simulink model "test_mdl_NI"  (R2018a)
settings: Solver=VariableStepAuto  StartTime=0.0  StopTime=10.0  RelTol=1e-3
(part 20 of 24)

== system test_mdl_NI/CAN_Signal/GWM/Other_GWMTx/PreCond_Hev_Data2_FD1 ==
  in : Inport
  BattTracClntFlw_Pc_Rq : Subsystem
  BattTrac_I_EstVsc : Subsystem
  DrvCondTpRrDefrs_B_Rq : Subsystem
  HtrnAin_UHi_Actl : Subsystem
  HtrnHvilOpen_B_Actl : Subsystem
  HtrnMil_D_Rq : Subsystem
  HtrnOvrTeLamp_B_Dsply : Subsystem
  HtrnSrvcRqd_B_Dsply : Subsystem
  PreCondActv_B_Actl : Subsystem
  PtWakeupDeltaT_T_Rq : Subsystem
  bus_creator : BusCreator  Inputs=10
  bus_selector : BusSelector  OutputSignals=BattTracClntFlw_Pc_Rq,BattTrac_I_EstVsc,DrvCondTpRrDefrs_B_Rq,HtrnAin_UHi_Actl,HtrnHvilOpen_B_Actl,HtrnMil_D_Rq,HtrnOvrTeLamp_B_Dsply,HtrnSrvcRqd_B_Dsply,PreCondActv_B_Actl,PtWakeupDeltaT_T_Rq
  out_port : Outport
  wires:
  bus_creator/1 -> out_port/1  "PreCond_Hev_Data2_FD1"
  BattTracClntFlw_Pc_Rq/1(out) -> bus_creator/1  "BattTracClntFlw_Pc_Rq"
  BattTrac_I_EstVsc/1(out) -> bus_creator/2  "BattTrac_I_EstVsc"
  DrvCondTpRrDefrs_B_Rq/1(out) -> bus_creator/3  "DrvCondTpRrDefrs_B_Rq"
  HtrnAin_UHi_Actl/1(out) -> bus_creator/4  "HtrnAin_UHi_Actl"
  HtrnHvilOpen_B_Actl/1(out) -> bus_creator/5  "HtrnHvilOpen_B_Actl"
  HtrnMil_D_Rq/1(out) -> bus_creator/6  "HtrnMil_D_Rq"
  HtrnOvrTeLamp_B_Dsply/1(out) -> bus_creator/7  "HtrnOvrTeLamp_B_Dsply"
  HtrnSrvcRqd_B_Dsply/1(out) -> bus_creator/8  "HtrnSrvcRqd_B_Dsply"
  PreCondActv_B_Actl/1(out) -> bus_creator/9  "PreCondActv_B_Actl"
  PtWakeupDeltaT_T_Rq/1(out) -> bus_creator/10  "PtWakeupDeltaT_T_Rq"
  bus_selector/1 -> BattTracClntFlw_Pc_Rq/1(in)  "<BattTracClntFlw_Pc_Rq>"
  bus_selector/2 -> BattTrac_I_EstVsc/1(in)  "<BattTrac_I_EstVsc>"
  bus_selector/3 -> DrvCondTpRrDefrs_B_Rq/1(in)  "<DrvCondTpRrDefrs_B_Rq>"
  bus_selector/4 -> HtrnAin_UHi_Actl/1(in)  "<HtrnAin_UHi_Actl>"
  bus_selector/5 -> HtrnHvilOpen_B_Actl/1(in)  "<HtrnHvilOpen_B_Actl>"
  bus_selector/6 -> HtrnMil_D_Rq/1(in)  "<HtrnMil_D_Rq>"
  bus_selector/7 -> HtrnOvrTeLamp_B_Dsply/1(in)  "<HtrnOvrTeLamp_B_Dsply>"
  bus_selector/8 -> HtrnSrvcRqd_B_Dsply/1(in)  "<HtrnSrvcRqd_B_Dsply>"
  bus_selector/9 -> PreCondActv_B_Actl/1(in)  "<PreCondActv_B_Actl>"
  bus_selector/10 -> PtWakeupDeltaT_T_Rq/1(in)  "<PtWakeupDeltaT_T_Rq>"
  in/1 -> bus_selector/1

== system test_mdl_NI/CAN_Signal/GWM/Other_GWMTx/Suspension_Data_FD1 ==
  in : Inport
  SuspClkSync_No_Rq : Subsystem
  SuspFrntRight_L_Actl : Subsystem
  SuspFrnt_L_Actl : Subsystem
  SuspFrnt_L_Prev : Subsystem
  SuspRearRight_L_Actl : Subsystem
  SuspRear_L_Actl : Subsystem
  SuspRear_L_Prev : Subsystem
  bus_creator : BusCreator  Inputs=7
  bus_selector : BusSelector  OutputSignals=SuspClkSync_No_Rq,SuspFrntRight_L_Actl,SuspFrnt_L_Actl,SuspFrnt_L_Prev,SuspRearRight_L_Actl,SuspRear_L_Actl,SuspRear_L_Prev
  out_port : Outport
  wires:
  bus_creator/1 -> out_port/1  "Suspension_Data_FD1"
  SuspClkSync_No_Rq/1(out) -> bus_creator/1  "SuspClkSync_No_Rq"
  SuspFrntRight_L_Actl/1(out) -> bus_creator/2  "SuspFrntRight_L_Actl"
  SuspFrnt_L_Actl/1(out) -> bus_creator/3  "SuspFrnt_L_Actl"
  SuspFrnt_L_Prev/1(out) -> bus_creator/4  "SuspFrnt_L_Prev"
  SuspRearRight_L_Actl/1(out) -> bus_creator/5  "SuspRearRight_L_Actl"
  SuspRear_L_Actl/1(out) -> bus_creator/6  "SuspRear_L_Actl"
  SuspRear_L_Prev/1(out) -> bus_creator/7  "SuspRear_L_Prev"
  bus_selector/1 -> SuspClkSync_No_Rq/1(in)  "<SuspClkSync_No_Rq>"
  bus_selector/2 -> SuspFrntRight_L_Actl/1(in)  "<SuspFrntRight_L_Actl>"
  bus_selector/3 -> SuspFrnt_L_Actl/1(in)  "<SuspFrnt_L_Actl>"
  bus_selector/4 -> SuspFrnt_L_Prev/1(in)  "<SuspFrnt_L_Prev>"
  bus_selector/5 -> SuspRearRight_L_Actl/1(in)  "<SuspRearRight_L_Actl>"
  bus_selector/6 -> SuspRear_L_Actl/1(in)  "<SuspRear_L_Actl>"
  bus_selector/7 -> SuspRear_L_Prev/1(in)  "<SuspRear_L_Prev>"
  in/1 -> bus_selector/1

== system test_mdl_NI/CAN_Signal/GWM/Other_GWMTx/TesterPhysicalResGWM_FD1 ==
  in : Inport
  TesterPhysicalResGWM_F1 : Subsystem
  bus_creator : BusCreator  Inputs=1
  bus_selector : BusSelector  OutputSignals=TesterPhysicalResGWM_F1
  out_port : Outport
  wires:
  bus_creator/1 -> out_port/1  "TesterPhysicalResGWM_FD1"
  TesterPhysicalResGWM_F1/1(out) -> bus_creator/1  "TesterPhysicalResGWM_F1"
  bus_selector/1 -> TesterPhysicalResGWM_F1/1(in)  "<TesterPhysicalResGWM_F1>"
  in/1 -> bus_selector/1

== system test_mdl_NI/CAN_Signal/GWM/Other_GWMTx/TrailerAid_Data_FD1 ==
  in : Inport
  TrlBrkInitOut_D_Rq : Subsystem
  TrlrAidEnbl_D_Rq : Subsystem
  TrlrAidSetup_D_Rq : Subsystem
  TrlrAnOffstDir_D_Mem : Subsystem
  TrlrAnOffst_An_Mem : Subsystem
  TrlrAxleToBmpr_L_Actl : Subsystem
  TrlrBallToBmpr_L_Actl : Subsystem
  TrlrId_No_Actl : Subsystem
  TrlrRvrseCancl_B_Rq : Subsystem
  TrlrTrgtOffst_L_Actl : Subsystem
  TrlrTrgtPtrnId_No_Mem : Subsystem
  TrlrTrgtToBmpr_L_Actl : Subsystem
  bus_creator : BusCreator  Inputs=12
  bus_selector : BusSelector  OutputSignals=TrlBrkInitOut_D_Rq,TrlrAidEnbl_D_Rq,TrlrAidSetup_D_Rq,TrlrAnOffstDir_D_Mem,TrlrAnOffst_An_Mem,TrlrAxleToBmpr_L_Actl,TrlrBallToBmpr_L_Actl,TrlrId_No_Actl,TrlrRvrseCancl_B_Rq,TrlrTrgtOffst_L_Actl,TrlrTrgtPtrnId_No_Mem,TrlrTrgtToBmpr_L_Actl
  out_port : Outport
  wires:
  bus_creator/1 -> out_port/1  "TrailerAid_Data_FD1"
  TrlBrkInitOut_D_Rq/1(out) -> bus_creator/1  "TrlBrkInitOut_D_Rq"
  TrlrAidEnbl_D_Rq/1(out) -> bus_creator/2  "TrlrAidEnbl_D_Rq"
  TrlrAidSetup_D_Rq/1(out) -> bus_creator/3  "TrlrAidSetup_D_Rq"
  TrlrAnOffstDir_D_Mem/1(out) -> bus_creator/4  "TrlrAnOffstDir_D_Mem"
  TrlrAnOffst_An_Mem/1(out) -> bus_creator/5  "TrlrAnOffst_An_Mem"
  TrlrAxleToBmpr_L_Actl/1(out) -> bus_creator/6  "TrlrAxleToBmpr_L_Actl"
  TrlrBallToBmpr_L_Actl/1(out) -> bus_creator/7  "TrlrBallToBmpr_L_Actl"
  TrlrId_No_Actl/1(out) -> bus_creator/8  "TrlrId_No_Actl"
  TrlrRvrseCancl_B_Rq/1(out) -> bus_creator/9  "TrlrRvrseCancl_B_Rq"
  TrlrTrgtOffst_L_Actl/1(out) -> bus_creator/10  "TrlrTrgtOffst_L_Actl"
  TrlrTrgtPtrnId_No_Mem/1(out) -> bus_creator/11  "TrlrTrgtPtrnId_No_Mem"
  TrlrTrgtToBmpr_L_Actl/1(out) -> bus_creator/12  "TrlrTrgtToBmpr_L_Actl"
  bus_selector/1 -> TrlBrkInitOut_D_Rq/1(in)  "<TrlBrkInitOut_D_Rq>"
  bus_selector/2 -> TrlrAidEnbl_D_Rq/1(in)  "<TrlrAidEnbl_D_Rq>"
  bus_selector/3 -> TrlrAidSetup_D_Rq/1(in)  "<TrlrAidSetup_D_Rq>"
  bus_selector/4 -> TrlrAnOffstDir_D_Mem/1(in)  "<TrlrAnOffstDir_D_Mem>"
  bus_selector/5 -> TrlrAnOffst_An_Mem/1(in)  "<TrlrAnOffst_An_Mem>"
  bus_selector/6 -> TrlrAxleToBmpr_L_Actl/1(in)  "<TrlrAxleToBmpr_L_Actl>"
  bus_selector/7 -> TrlrBallToBmpr_L_Actl/1(in)  "<TrlrBallToBmpr_L_Actl>"
  bus_selector/8 -> TrlrId_No_Actl/1(in)  "<TrlrId_No_Actl>"
  bus_selector/9 -> TrlrRvrseCancl_B_Rq/1(in)  "<TrlrRvrseCancl_B_Rq>"
  bus_selector/10 -> TrlrTrgtOffst_L_Actl/1(in)  "<TrlrTrgtOffst_L_Actl>"
  bus_selector/11 -> TrlrTrgtPtrnId_No_Mem/1(in)  "<TrlrTrgtPtrnId_No_Mem>"
  bus_selector/12 -> TrlrTrgtToBmpr_L_Actl/1(in)  "<TrlrTrgtToBmpr_L_Actl>"
  in/1 -> bus_selector/1

== system test_mdl_NI/CAN_Signal/GWM/Other_GWMTx/TrailerAid_Stat1_FD1 ==
  in : Inport
  TrlrSnsId_No_Actl : Subsystem
  bus_creator : BusCreator  Inputs=1
  bus_selector : BusSelector  OutputSignals=TrlrSnsId_No_Actl
  out_port : Outport
  wires:
  bus_creator/1 -> out_port/1  "TrailerAid_Stat1_FD1"
  TrlrSnsId_No_Actl/1(out) -> bus_creator/1  "TrlrSnsId_No_Actl"
  bus_selector/1 -> TrlrSnsId_No_Actl/1(in)  "<TrlrSnsId_No_Actl>"
  in/1 -> bus_selector/1

== system test_mdl_NI/CAN_Signal/GWM/Other_GWMTx/TrailerAid_Stat2_FD1 ==
  in : Inport
  TrlrHitYaw_AnRate_Actl : Subsystem
  TrlrHitchYaw_An_Actl : Subsystem
  TrlrHitchYaw_D_Stat : Subsystem
  TrlrYawWActl_D_Qf : Subsystem
  TrlrYaw_W_Actl : Subsystem
  bus_creator : BusCreator  Inputs=5
  bus_selector : BusSelector  OutputSignals=TrlrHitYaw_AnRate_Actl,TrlrHitchYaw_An_Actl,TrlrHitchYaw_D_Stat,TrlrYawWActl_D_Qf,TrlrYaw_W_Actl
  out_port : Outport
  wires:
  bus_creator/1 -> out_port/1  "TrailerAid_Stat2_FD1"
  TrlrHitYaw_AnRate_Actl/1(out) -> bus_creator/1  "TrlrHitYaw_AnRate_Actl"
  TrlrHitchYaw_An_Actl/1(out) -> bus_creator/2  "TrlrHitchYaw_An_Actl"
  TrlrHitchYaw_D_Stat/1(out) -> bus_creator/3  "TrlrHitchYaw_D_Stat"
  TrlrYawWActl_D_Qf/1(out) -> bus_creator/4  "TrlrYawWActl_D_Qf"
  TrlrYaw_W_Actl/1(out) -> bus_creator/5  "TrlrYaw_W_Actl"
  bus_selector/1 -> TrlrHitYaw_AnRate_Actl/1(in)  "<TrlrHitYaw_AnRate_Actl>"
  bus_selector/2 -> TrlrHitchYaw_An_Actl/1(in)  "<TrlrHitchYaw_An_Actl>"
  bus_selector/3 -> TrlrHitchYaw_D_Stat/1(in)  "<TrlrHitchYaw_D_Stat>"
  bus_selector/4 -> TrlrYawWActl_D_Qf/1(in)  "<TrlrYawWActl_D_Qf>"
  bus_selector/5 -> TrlrYaw_W_Actl/1(in)  "<TrlrYaw_W_Actl>"
  in/1 -> bus_selector/1

== system test_mdl_NI/CAN_Signal/GWM/Other_GWMTx/TrailerBrakeInfo_FD1 ==
  in : Inport
  StopLamp_B_RqTrlrBrk : Subsystem
  TrlBrkInitOut_D_Stat : Subsystem
  TrlrBrkActCirct_B_Falt : Subsystem
  TrlrBrkActCnnct_B_Actl : Subsystem
  TrlrBrkCtl_B_Falt : Subsystem
  TrlrBrkDcnnt_B_Actl : Subsystem
  TrlrBrkDsply_B_Rq : Subsystem
  TrlrBrkGain_No_Actl : Subsystem
  TrlrBrkMde_D_Actl : Subsystem
  TrlrBrkOut_No_Dsply : Subsystem
  bus_creator : BusCreator  Inputs=10
  bus_selector : BusSelector  OutputSignals=StopLamp_B_RqTrlrBrk,TrlBrkInitOut_D_Stat,TrlrBrkActCirct_B_Falt,TrlrBrkActCnnct_B_Actl,TrlrBrkCtl_B_Falt,TrlrBrkDcnnt_B_Actl,TrlrBrkDsply_B_Rq,TrlrBrkGain_No_Actl,TrlrBrkMde_D_Actl,TrlrBrkOut_No_Dsply
  out_port : Outport
  wires:
  bus_creator/1 -> out_port/1  "TrailerBrakeInfo_FD1"
  StopLamp_B_RqTrlrBrk/1(out) -> bus_creator/1  "StopLamp_B_RqTrlrBrk"
  TrlBrkInitOut_D_Stat/1(out) -> bus_creator/2  "TrlBrkInitOut_D_Stat"
  TrlrBrkActCirct_B_Falt/1(out) -> bus_creator/3  "TrlrBrkActCirct_B_Falt"
  TrlrBrkActCnnct_B_Actl/1(out) -> bus_creator/4  "TrlrBrkActCnnct_B_Actl"
  TrlrBrkCtl_B_Falt/1(out) -> bus_creator/5  "TrlrBrkCtl_B_Falt"
  TrlrBrkDcnnt_B_Actl/1(out) -> bus_creator/6  "TrlrBrkDcnnt_B_Actl"
  TrlrBrkDsply_B_Rq/1(out) -> bus_creator/7  "TrlrBrkDsply_B_Rq"
  TrlrBrkGain_No_Actl/1(out) -> bus_creator/8  "TrlrBrkGain_No_Actl"
  TrlrBrkMde_D_Actl/1(out) -> bus_creator/9  "TrlrBrkMde_D_Actl"
  TrlrBrkOut_No_Dsply/1(out) -> bus_creator/10  "TrlrBrkOut_No_Dsply"
  bus_selector/1 -> StopLamp_B_RqTrlrBrk/1(in)  "<StopLamp_B_RqTrlrBrk>"
  bus_selector/2 -> TrlBrkInitOut_D_Stat/1(in)  "<TrlBrkInitOut_D_Stat>"
  bus_selector/3 -> TrlrBrkActCirct_B_Falt/1(in)  "<TrlrBrkActCirct_B_Falt>"
  bus_selector/4 -> TrlrBrkActCnnct_B_Actl/1(in)  "<TrlrBrkActCnnct_B_Actl>"
  bus_selector/5 -> TrlrBrkCtl_B_Falt/1(in)  "<TrlrBrkCtl_B_Falt>"
  bus_selector/6 -> TrlrBrkDcnnt_B_Actl/1(in)  "<TrlrBrkDcnnt_B_Actl>"
  bus_selector/7 -> TrlrBrkDsply_B_Rq/1(in)  "<TrlrBrkDsply_B_Rq>"
  bus_selector/8 -> TrlrBrkGain_No_Actl/1(in)  "<TrlrBrkGain_No_Actl>"
  bus_selector/9 -> TrlrBrkMde_D_Actl/1(in)  "<TrlrBrkMde_D_Actl>"
  bus_selector/10 -> TrlrBrkOut_No_Dsply/1(in)  "<TrlrBrkOut_No_Dsply>"
  in/1 -> bus_selector/1

== system test_mdl_NI/CAN_Signal/GWM/Other_GWMTx/TrailerInfo_2_FD1 ==
  in : Inport
  TrlrAidAn_URate_Actl : Subsystem
  TrlrAidAn_U_Actl : Subsystem
  TrlrAidCtl_U_RqDrv : Subsystem
  TrlrAidSwtch_D_RqDrv : Subsystem
  bus_creator : BusCreator  Inputs=4
  bus_selector : BusSelector  OutputSignals=TrlrAidAn_URate_Actl,TrlrAidAn_U_Actl,TrlrAidCtl_U_RqDrv,TrlrAidSwtch_D_RqDrv
  out_port : Outport
  wires:
  bus_creator/1 -> out_port/1  "TrailerInfo_2_FD1"
  TrlrAidAn_URate_Actl/1(out) -> bus_creator/1  "TrlrAidAn_URate_Actl"
  TrlrAidAn_U_Actl/1(out) -> bus_creator/2  "TrlrAidAn_U_Actl"
  TrlrAidCtl_U_RqDrv/1(out) -> bus_creator/3  "TrlrAidCtl_U_RqDrv"
  TrlrAidSwtch_D_RqDrv/1(out) -> bus_creator/4  "TrlrAidSwtch_D_RqDrv"
  bus_selector/1 -> TrlrAidAn_URate_Actl/1(in)  "<TrlrAidAn_URate_Actl>"
  bus_selector/2 -> TrlrAidAn_U_Actl/1(in)  "<TrlrAidAn_U_Actl>"
  bus_selector/3 -> TrlrAidCtl_U_RqDrv/1(in)  "<TrlrAidCtl_U_RqDrv>"
  bus_selector/4 -> TrlrAidSwtch_D_RqDrv/1(in)  "<TrlrAidSwtch_D_RqDrv>"
  in/1 -> bus_selector/1

== system test_mdl_NI/CAN_Signal/GWM/Other_GWMTx/TrailerInfo_FD1 ==
  in : Inport
  ParkLampTrlrOut_B_Stat : Subsystem
  StopLampTrlrOut_B_Stat : Subsystem
  TrlrBattChrg_D_Stat : Subsystem
  TrlrLampCnnct_B_Actl : Subsystem
  TrlrLampCtl_D_Stat : Subsystem
  TurnLampTrlrRl_B_Stat : Subsystem
  TurnLampTrlrRr_B_Stat : Subsystem
  bus_creator : BusCreator  Inputs=7
  bus_selector : BusSelector  OutputSignals=ParkLampTrlrOut_B_Stat,StopLampTrlrOut_B_Stat,TrlrBattChrg_D_Stat,TrlrLampCnnct_B_Actl,TrlrLampCtl_D_Stat,TurnLampTrlrRl_B_Stat,TurnLampTrlrRr_B_Stat
  out_port : Outport
  wires:
  bus_creator/1 -> out_port/1  "TrailerInfo_FD1"
  ParkLampTrlrOut_B_Stat/1(out) -> bus_creator/1  "ParkLampTrlrOut_B_Stat"
  StopLampTrlrOut_B_Stat/1(out) -> bus_creator/2  "StopLampTrlrOut_B_Stat"
  TrlrBattChrg_D_Stat/1(out) -> bus_creator/3  "TrlrBattChrg_D_Stat"
  TrlrLampCnnct_B_Actl/1(out) -> bus_creator/4  "TrlrLampCnnct_B_Actl"
  TrlrLampCtl_D_Stat/1(out) -> bus_creator/5  "TrlrLampCtl_D_Stat"
  TurnLampTrlrRl_B_Stat/1(out) -> bus_creator/6  "TurnLampTrlrRl_B_Stat"
  TurnLampTrlrRr_B_Stat/1(out) -> bus_creator/7  "TurnLampTrlrRr_B_Stat"
  bus_selector/1 -> ParkLampTrlrOut_B_Stat/1(in)  "<ParkLampTrlrOut_B_Stat>"
  bus_selector/2 -> StopLampTrlrOut_B_Stat/1(in)  "<StopLampTrlrOut_B_Stat>"
  bus_selector/3 -> TrlrBattChrg_D_Stat/1(in)  "<TrlrBattChrg_D_Stat>"
  bus_selector/4 -> TrlrLampCnnct_B_Actl/1(in)  "<TrlrLampCnnct_B_Actl>"
  bus_selector/5 -> TrlrLampCtl_D_Stat/1(in)  "<TrlrLampCtl_D_Stat>"
  bus_selector/6 -> TurnLampTrlrRl_B_Stat/1(in)  "<TurnLampTrlrRl_B_Stat>"
  bus_selector/7 -> TurnLampTrlrRr_B_Stat/1(in)  "<TurnLampTrlrRr_B_Stat>"
  in/1 -> bus_selector/1

== system test_mdl_NI/CAN_Signal/GWM/Other_GWMTx/VeyDynamics_Data_FD1 ==
  in : Inport
  AdptDrvMdeChassis_D_Rq : Subsystem
  AdptDrvMdePt_D_Rq : Subsystem
  AirSprngRateFl_D_Rq : Subsystem
  AirSprngRateFr_D_Rq : Subsystem
  AirSprngRateRl_D_Rq : Subsystem
  AirSprngRateRr_D_Rq : Subsystem
  AirSuspMsgTxt_D_Rq : Subsystem
  AirSusp_D_Stat : Subsystem
  BrkPadMsgTxt_D_Rq : Subsystem
  CcdMsgTxt_D_RqDsply : Subsystem
  Ccd_B_Falt : Subsystem
  SelDrvMdeSusp_D_Stat : Subsystem
  SuspDrvMde_D_Stat : Subsystem
  SuspType_B_Stat : Subsystem
  SuspVLim_B_Rq : Subsystem
  bus_creator : BusCreator  Inputs=15
  bus_selector : BusSelector  OutputSignals=AdptDrvMdeChassis_D_Rq,AdptDrvMdePt_D_Rq,AirSprngRateFl_D_Rq,AirSprngRateFr_D_Rq,AirSprngRateRl_D_Rq,AirSprngRateRr_D_Rq,AirSuspMsgTxt_D_Rq,AirSusp_D_Stat,BrkPadMsgTxt_D_Rq,CcdMsgTxt_D_RqDsply,Ccd_B_Falt,SelDrvMdeSusp_D_Stat,SuspDrvMde_D_Stat,SuspType_B_Stat,SuspVLim_B_Rq
  out_port : Outport
  wires:
  bus_creator/1 -> out_port/1  "VeyDynamics_Data_FD1"
  AdptDrvMdeChassis_D_Rq/1(out) -> bus_creator/1  "AdptDrvMdeChassis_D_Rq"
  AdptDrvMdePt_D_Rq/1(out) -> bus_creator/2  "AdptDrvMdePt_D_Rq"
  AirSprngRateFl_D_Rq/1(out) -> bus_creator/3  "AirSprngRateFl_D_Rq"
  AirSprngRateFr_D_Rq/1(out) -> bus_creator/4  "AirSprngRateFr_D_Rq"
  AirSprngRateRl_D_Rq/1(out) -> bus_creator/5  "AirSprngRateRl_D_Rq"
  AirSprngRateRr_D_Rq/1(out) -> bus_creator/6  "AirSprngRateRr_D_Rq"
  AirSuspMsgTxt_D_Rq/1(out) -> bus_creator/7  "AirSuspMsgTxt_D_Rq"
  AirSusp_D_Stat/1(out) -> bus_creator/8  "AirSusp_D_Stat"
  BrkPadMsgTxt_D_Rq/1(out) -> bus_creator/9  "BrkPadMsgTxt_D_Rq"
  CcdMsgTxt_D_RqDsply/1(out) -> bus_creator/10  "CcdMsgTxt_D_RqDsply"
  Ccd_B_Falt/1(out) -> bus_creator/11  "Ccd_B_Falt"
  SelDrvMdeSusp_D_Stat/1(out) -> bus_creator/12  "SelDrvMdeSusp_D_Stat"
  SuspDrvMde_D_Stat/1(out) -> bus_creator/13  "SuspDrvMde_D_Stat"
  SuspType_B_Stat/1(out) -> bus_creator/14  "SuspType_B_Stat"
  SuspVLim_B_Rq/1(out) -> bus_creator/15  "SuspVLim_B_Rq"
  bus_selector/1 -> AdptDrvMdeChassis_D_Rq/1(in)  "<AdptDrvMdeChassis_D_Rq>"
  bus_selector/2 -> AdptDrvMdePt_D_Rq/1(in)  "<AdptDrvMdePt_D_Rq>"
  bus_selector/3 -> AirSprngRateFl_D_Rq/1(in)  "<AirSprngRateFl_D_Rq>"
  bus_selector/4 -> AirSprngRateFr_D_Rq/1(in)  "<AirSprngRateFr_D_Rq>"
  bus_selector/5 -> AirSprngRateRl_D_Rq/1(in)  "<AirSprngRateRl_D_Rq>"
  bus_selector/6 -> AirSprngRateRr_D_Rq/1(in)  "<AirSprngRateRr_D_Rq>"
  bus_selector/7 -> AirSuspMsgTxt_D_Rq/1(in)  "<AirSuspMsgTxt_D_Rq>"
  bus_selector/8 -> AirSusp_D_Stat/1(in)  "<AirSusp_D_Stat>"
  bus_selector/9 -> BrkPadMsgTxt_D_Rq/1(in)  "<BrkPadMsgTxt_D_Rq>"
  bus_selector/10 -> CcdMsgTxt_D_RqDsply/1(in)  "<CcdMsgTxt_D_RqDsply>"
  bus_selector/11 -> Ccd_B_Falt/1(in)  "<Ccd_B_Falt>"
  bus_selector/12 -> SelDrvMdeSusp_D_Stat/1(in)  "<SelDrvMdeSusp_D_Stat>"
  bus_selector/13 -> SuspDrvMde_D_Stat/1(in)  "<SuspDrvMde_D_Stat>"
  bus_selector/14 -> SuspType_B_Stat/1(in)  "<SuspType_B_Stat>"
  bus_selector/15 -> SuspVLim_B_Rq/1(in)  "<SuspVLim_B_Rq>"
  in/1 -> bus_selector/1

== system test_mdl_NI/CAN_Signal/GWM/RCM/RCMSerialNumber_FD1_454 ==
  in : Inport
  RCMSerialNoByte1 : Subsystem
  RCMSerialNoByte2 : Subsystem
  RCMSerialNoByte3 : Subsystem
  RCMSerialNoByte4 : Subsystem
  RCMSerialNoByte5 : Subsystem
  RCMSerialNoByte6 : Subsystem
  RCMSerialNoByte7 : Subsystem
  RCMSerialNoByte8 : Subsystem
  bus_creator : BusCreator  Inputs=8
  bus_selector : BusSelector  OutputSignals=RCMSerialNoByte1,RCMSerialNoByte2,RCMSerialNoByte3,RCMSerialNoByte4,RCMSerialNoByte5,RCMSerialNoByte6,RCMSerialNoByte7,RCMSerialNoByte8
  out_port : Outport
  wires:
  bus_creator/1 -> out_port/1  "RCMSerialNumber_FD1_454"
  RCMSerialNoByte1/1(out) -> bus_creator/1  "RCMSerialNoByte1"
  RCMSerialNoByte2/1(out) -> bus_creator/2  "RCMSerialNoByte2"
  RCMSerialNoByte3/1(out) -> bus_creator/3  "RCMSerialNoByte3"
  RCMSerialNoByte4/1(out) -> bus_creator/4  "RCMSerialNoByte4"
  RCMSerialNoByte5/1(out) -> bus_creator/5  "RCMSerialNoByte5"
  RCMSerialNoByte6/1(out) -> bus_creator/6  "RCMSerialNoByte6"
  RCMSerialNoByte7/1(out) -> bus_creator/7  "RCMSerialNoByte7"
  RCMSerialNoByte8/1(out) -> bus_creator/8  "RCMSerialNoByte8"
  bus_selector/1 -> RCMSerialNoByte1/1(in)  "<RCMSerialNoByte1>"
  bus_selector/2 -> RCMSerialNoByte2/1(in)  "<RCMSerialNoByte2>"
  bus_selector/3 -> RCMSerialNoByte3/1(in)  "<RCMSerialNoByte3>"
  bus_selector/4 -> RCMSerialNoByte4/1(in)  "<RCMSerialNoByte4>"
  bus_selector/5 -> RCMSerialNoByte5/1(in)  "<RCMSerialNoByte5>"
  bus_selector/6 -> RCMSerialNoByte6/1(in)  "<RCMSerialNoByte6>"
  bus_selector/7 -> RCMSerialNoByte7/1(in)  "<RCMSerialNoByte7>"
  bus_selector/8 -> RCMSerialNoByte8/1(in)  "<RCMSerialNoByte8>"
  in/1 -> bus_selector/1

== system test_mdl_NI/CAN_Signal/GWM/RCM/RCMStatusMessage2_FD1_4C ==
  in : Inport
  EDRTriggerEvntSync : Subsystem
  FirstRowBuckleDriver : Subsystem
  FirstRowBuckleMid : Subsystem
  FirstRowBucklePsngr : Subsystem
  PassRstrnInd_Req : Subsystem
  PsngrFmidDetct_D_Actl : Subsystem
  PsngrFrntDetct_D_Actl : Subsystem
  RILReq : Subsystem
  RstrnImpactEvntStatus : Subsystem
  RstrnPsngrOn_D_Stat : Subsystem
  SecondRowBuckleDriver : Subsystem
  SecondRowBuckleMid : Subsystem
  SecondRowBucklePsngr : Subsystem
  ThirdRowBuckleDriver : Subsystem
  ThirdRowBuckleMid : Subsystem
  ThirdRowBucklePsngr : Subsystem
  bus_creator : BusCreator  Inputs=16
  bus_selector : BusSelector  OutputSignals=EDRTriggerEvntSync,FirstRowBuckleDriver,FirstRowBuckleMid,FirstRowBucklePsngr,PassRstrnInd_Req,PsngrFmidDetct_D_Actl,PsngrFrntDetct_D_Actl,RILReq,RstrnImpactEvntStatus,RstrnPsngrOn_D_Stat,SecondRowBuckleDriver,SecondRowBuckleMid,SecondRowBucklePsngr,ThirdRowBuckleDriver,ThirdRowBuckleMid,ThirdRowBucklePsngr
  out_port : Outport
  wires:
  bus_creator/1 -> out_port/1  "RCMStatusMessage2_FD1_4C"
  EDRTriggerEvntSync/1(out) -> bus_creator/1  "EDRTriggerEvntSync"
  FirstRowBuckleDriver/1(out) -> bus_creator/2  "FirstRowBuckleDriver"
  FirstRowBuckleMid/1(out) -> bus_creator/3  "FirstRowBuckleMid"
  FirstRowBucklePsngr/1(out) -> bus_creator/4  "FirstRowBucklePsngr"
  PassRstrnInd_Req/1(out) -> bus_creator/5  "PassRstrnInd_Req"
  PsngrFmidDetct_D_Actl/1(out) -> bus_creator/6  "PsngrFmidDetct_D_Actl"
  PsngrFrntDetct_D_Actl/1(out) -> bus_creator/7  "PsngrFrntDetct_D_Actl"
  RILReq/1(out) -> bus_creator/8  "RILReq"
  RstrnImpactEvntStatus/1(out) -> bus_creator/9  "RstrnImpactEvntStatus"
  RstrnPsngrOn_D_Stat/1(out) -> bus_creator/10  "RstrnPsngrOn_D_Stat"
  SecondRowBuckleDriver/1(out) -> bus_creator/11  "SecondRowBuckleDriver"
  SecondRowBuckleMid/1(out) -> bus_creator/12  "SecondRowBuckleMid"
  SecondRowBucklePsngr/1(out) -> bus_creator/13  "SecondRowBucklePsngr"
  ThirdRowBuckleDriver/1(out) -> bus_creator/14  "ThirdRowBuckleDriver"
  ThirdRowBuckleMid/1(out) -> bus_creator/15  "ThirdRowBuckleMid"
  ThirdRowBucklePsngr/1(out) -> bus_creator/16  "ThirdRowBucklePsngr"
  bus_selector/1 -> EDRTriggerEvntSync/1(in)  "<EDRTriggerEvntSync>"
  bus_selector/2 -> FirstRowBuckleDriver/1(in)  "<FirstRowBuckleDriver>"
  bus_selector/3 -> FirstRowBuckleMid/1(in)  "<FirstRowBuckleMid>"
  bus_selector/4 -> FirstRowBucklePsngr/1(in)  "<FirstRowBucklePsngr>"
  bus_selector/5 -> PassRstrnInd_Req/1(in)  "<PassRstrnInd_Req>"
  bus_selector/6 -> PsngrFmidDetct_D_Actl/1(in)  "<PsngrFmidDetct_D_Actl>"
  bus_selector/7 -> PsngrFrntDetct_D_Actl/1(in)  "<PsngrFrntDetct_D_Actl>"
  bus_selector/8 -> RILReq/1(in)  "<RILReq>"
  bus_selector/9 -> RstrnImpactEvntStatus/1(in)  "<RstrnImpactEvntStatus>"
  bus_selector/10 -> RstrnPsngrOn_D_Stat/1(in)  "<RstrnPsngrOn_D_Stat>"
  bus_selector/11 -> SecondRowBuckleDriver/1(in)  "<SecondRowBuckleDriver>"
  bus_selector/12 -> SecondRowBuckleMid/1(in)  "<SecondRowBuckleMid>"
  bus_selector/13 -> SecondRowBucklePsngr/1(in)  "<SecondRowBucklePsngr>"
  bus_selector/14 -> ThirdRowBuckleDriver/1(in)  "<ThirdRowBuckleDriver>"
  bus_selector/15 -> ThirdRowBuckleMid/1(in)  "<ThirdRowBuckleMid>"
  bus_selector/16 -> ThirdRowBucklePsngr/1(in)  "<ThirdRowBucklePsngr>"
  in/1 -> bus_selector/1

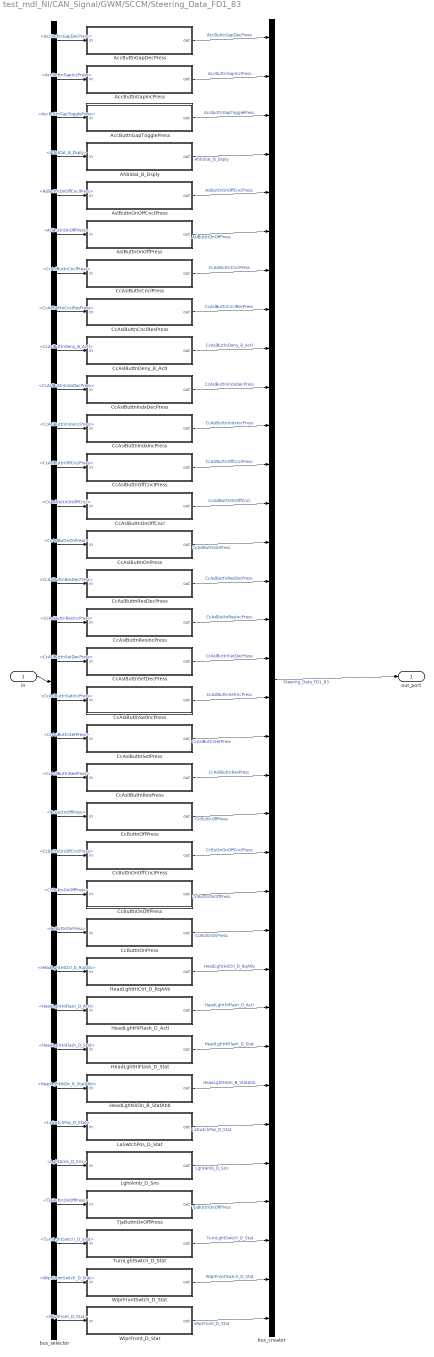
== system test_mdl_NI/CAN_Signal/GWM/SCCM/Steering_Data_FD1_83 ==
  in : Inport
  AccButtnGapDecPress : Subsystem
  AccButtnGapIncPress : Subsystem
  AccButtnGapTogglePress : Subsystem
  AhbStat_B_Dsply : Subsystem
  AslButtnOnOffCnclPress : Subsystem
  AslButtnOnOffPress : Subsystem
  CcAslButtnCnclPress : Subsystem
  CcAslButtnCnclResPress : Subsystem
  CcAslButtnDeny_B_Actl : Subsystem
  CcAslButtnIndxDecPress : Subsystem
  CcAslButtnIndxIncPress : Subsystem
  CcAslButtnOffCnclPress : Subsystem
  CcAslButtnOnOffCncl : Subsystem
  CcAslButtnOnPress : Subsystem
  CcAslButtnResDecPress : Subsystem
  CcAslButtnResIncPress : Subsystem
  CcAslButtnSetDecPress : Subsystem
  CcAslButtnSetIncPress : Subsystem
  CcAslButtnSetPress : Subsystem
  CcAsllButtnResPress : Subsystem
  CcButtnOffPress : Subsystem
  CcButtnOnOffCnclPress : Subsystem
  CcButtnOnOffPress : Subsystem
  CcButtnOnPress : Subsystem
  HeadLghtHiCtrl_D_RqAhb : Subsystem
  HeadLghtHiFlash_D_Actl : Subsystem
  HeadLghtHiFlash_D_Stat : Subsystem
  HeadLghtHiOn_B_StatAhb : Subsystem
  LaSwtchPos_D_Stat : Subsystem
  LghtAmb_D_Sns : Subsystem
  TjaButtnOnOffPress : Subsystem
  TurnLghtSwtch_D_Stat : Subsystem
  WiprFrontSwtch_D_Stat : Subsystem
  WiprFront_D_Stat : Subsystem
  bus_creator : BusCreator  Inputs=34
  bus_selector : BusSelector  OutputSignals=AccButtnGapDecPress,AccButtnGapIncPress,AccButtnGapTogglePress,AhbStat_B_Dsply,AslButtnOnOffCnclPress,AslButtnOnOffPress,CcAslButtnCnclPress,CcAslButtnCnclResPress,CcAslButtnDeny_B_Actl,CcAslButtnIndxDecPress,CcAslButtnIndxIncPress,CcAslButtnOffCnclPress,CcAslButtnOnOffCncl,CcAslButtnOnPress,CcAslButtnResDecPress,CcAslButtnResIncPress,CcAslButtnSetDecPress,CcAslButtnSetIncPress,CcAslButtnSetPress,CcAsllButtnResPress,CcButtnOffPress,CcButtnOnOffCnclPress,CcButtnOnOffPress,CcButtnOnPress,HeadLghtHiCtrl_D_RqAhb,HeadLghtHiFlash_D_Actl,HeadLghtHiFlash_D_Stat,HeadLghtHiOn_B_StatAhb,LaSwtchPos_D_Stat,LghtAmb_D_Sns,TjaButtnOnOffPress,TurnLghtSwtch_D_Stat,WiprFrontSwtch_D_Stat,WiprFront_D_Stat
  out_port : Outport
  wires:
  bus_creator/1 -> out_port/1  "Steering_Data_FD1_83"
  AccButtnGapDecPress/1(out) -> bus_creator/1  "AccButtnGapDecPress"
  AccButtnGapIncPress/1(out) -> bus_creator/2  "AccButtnGapIncPress"
  AccButtnGapTogglePress/1(out) -> bus_creator/3  "AccButtnGapTogglePress"
  AhbStat_B_Dsply/1(out) -> bus_creator/4  "AhbStat_B_Dsply"
  AslButtnOnOffCnclPress/1(out) -> bus_creator/5  "AslButtnOnOffCnclPress"
  AslButtnOnOffPress/1(out) -> bus_creator/6  "AslButtnOnOffPress"
  CcAslButtnCnclPress/1(out) -> bus_creator/7  "CcAslButtnCnclPress"
  CcAslButtnCnclResPress/1(out) -> bus_creator/8  "CcAslButtnCnclResPress"
  CcAslButtnDeny_B_Actl/1(out) -> bus_creator/9  "CcAslButtnDeny_B_Actl"
  CcAslButtnIndxDecPress/1(out) -> bus_creator/10  "CcAslButtnIndxDecPress"
  CcAslButtnIndxIncPress/1(out) -> bus_creator/11  "CcAslButtnIndxIncPress"
  CcAslButtnOffCnclPress/1(out) -> bus_creator/12  "CcAslButtnOffCnclPress"
  CcAslButtnOnOffCncl/1(out) -> bus_creator/13  "CcAslButtnOnOffCncl"
  CcAslButtnOnPress/1(out) -> bus_creator/14  "CcAslButtnOnPress"
  CcAslButtnResDecPress/1(out) -> bus_creator/15  "CcAslButtnResDecPress"
  CcAslButtnResIncPress/1(out) -> bus_creator/16  "CcAslButtnResIncPress"
  CcAslButtnSetDecPress/1(out) -> bus_creator/17  "CcAslButtnSetDecPress"
  CcAslButtnSetIncPress/1(out) -> bus_creator/18  "CcAslButtnSetIncPress"
  CcAslButtnSetPress/1(out) -> bus_creator/19  "CcAslButtnSetPress"
  CcAsllButtnResPress/1(out) -> bus_creator/20  "CcAsllButtnResPress"
  CcButtnOffPress/1(out) -> bus_creator/21  "CcButtnOffPress"
  CcButtnOnOffCnclPress/1(out) -> bus_creator/22  "CcButtnOnOffCnclPress"
  CcButtnOnOffPress/1(out) -> bus_creator/23  "CcButtnOnOffPress"
  CcButtnOnPress/1(out) -> bus_creator/24  "CcButtnOnPress"
  HeadLghtHiCtrl_D_RqAhb/1(out) -> bus_creator/25  "HeadLghtHiCtrl_D_RqAhb"
  HeadLghtHiFlash_D_Actl/1(out) -> bus_creator/26  "HeadLghtHiFlash_D_Actl"
  HeadLghtHiFlash_D_Stat/1(out) -> bus_creator/27  "HeadLghtHiFlash_D_Stat"
  HeadLghtHiOn_B_StatAhb/1(out) -> bus_creator/28  "HeadLghtHiOn_B_StatAhb"
  LaSwtchPos_D_Stat/1(out) -> bus_creator/29  "LaSwtchPos_D_Stat"
  LghtAmb_D_Sns/1(out) -> bus_creator/30  "LghtAmb_D_Sns"
  TjaButtnOnOffPress/1(out) -> bus_creator/31  "TjaButtnOnOffPress"
  TurnLghtSwtch_D_Stat/1(out) -> bus_creator/32  "TurnLghtSwtch_D_Stat"
  WiprFrontSwtch_D_Stat/1(out) -> bus_creator/33  "WiprFrontSwtch_D_Stat"
  WiprFront_D_Stat/1(out) -> bus_creator/34  "WiprFront_D_Stat"
  bus_selector/1 -> AccButtnGapDecPress/1(in)  "<AccButtnGapDecPress>"
  bus_selector/2 -> AccButtnGapIncPress/1(in)  "<AccButtnGapIncPress>"
  bus_selector/3 -> AccButtnGapTogglePress/1(in)  "<AccButtnGapTogglePress>"
  bus_selector/4 -> AhbStat_B_Dsply/1(in)  "<AhbStat_B_Dsply>"
  bus_selector/5 -> AslButtnOnOffCnclPress/1(in)  "<AslButtnOnOffCnclPress>"
  bus_selector/6 -> AslButtnOnOffPress/1(in)  "<AslButtnOnOffPress>"
  bus_selector/7 -> CcAslButtnCnclPress/1(in)  "<CcAslButtnCnclPress>"
  bus_selector/8 -> CcAslButtnCnclResPress/1(in)  "<CcAslButtnCnclResPress>"
  bus_selector/9 -> CcAslButtnDeny_B_Actl/1(in)  "<CcAslButtnDeny_B_Actl>"
  bus_selector/10 -> CcAslButtnIndxDecPress/1(in)  "<CcAslButtnIndxDecPress>"
  bus_selector/11 -> CcAslButtnIndxIncPress/1(in)  "<CcAslButtnIndxIncPress>"
  bus_selector/12 -> CcAslButtnOffCnclPress/1(in)  "<CcAslButtnOffCnclPress>"
  bus_selector/13 -> CcAslButtnOnOffCncl/1(in)  "<CcAslButtnOnOffCncl>"
  bus_selector/14 -> CcAslButtnOnPress/1(in)  "<CcAslButtnOnPress>"
  bus_selector/15 -> CcAslButtnResDecPress/1(in)  "<CcAslButtnResDecPress>"
  bus_selector/16 -> CcAslButtnResIncPress/1(in)  "<CcAslButtnResIncPress>"
  bus_selector/17 -> CcAslButtnSetDecPress/1(in)  "<CcAslButtnSetDecPress>"
  bus_selector/18 -> CcAslButtnSetIncPress/1(in)  "<CcAslButtnSetIncPress>"
  bus_selector/19 -> CcAslButtnSetPress/1(in)  "<CcAslButtnSetPress>"
  bus_selector/20 -> CcAsllButtnResPress/1(in)  "<CcAsllButtnResPress>"
  bus_selector/21 -> CcButtnOffPress/1(in)  "<CcButtnOffPress>"
  bus_selector/22 -> CcButtnOnOffCnclPress/1(in)  "<CcButtnOnOffCnclPress>"
  bus_selector/23 -> CcButtnOnOffPress/1(in)  "<CcButtnOnOffPress>"
  bus_selector/24 -> CcButtnOnPress/1(in)  "<CcButtnOnPress>"
  bus_selector/25 -> HeadLghtHiCtrl_D_RqAhb/1(in)  "<HeadLghtHiCtrl_D_RqAhb>"
  bus_selector/26 -> HeadLghtHiFlash_D_Actl/1(in)  "<HeadLghtHiFlash_D_Actl>"
  bus_selector/27 -> HeadLghtHiFlash_D_Stat/1(in)  "<HeadLghtHiFlash_D_Stat>"
  bus_selector/28 -> HeadLghtHiOn_B_StatAhb/1(in)  "<HeadLghtHiOn_B_StatAhb>"
  bus_selector/29 -> LaSwtchPos_D_Stat/1(in)  "<LaSwtchPos_D_Stat>"
  bus_selector/30 -> LghtAmb_D_Sns/1(in)  "<LghtAmb_D_Sns>"
  bus_selector/31 -> TjaButtnOnOffPress/1(in)  "<TjaButtnOnOffPress>"
  bus_selector/32 -> TurnLghtSwtch_D_Stat/1(in)  "<TurnLghtSwtch_D_Stat>"
  bus_selector/33 -> WiprFrontSwtch_D_Stat/1(in)  "<WiprFrontSwtch_D_Stat>"
  bus_selector/34 -> WiprFront_D_Stat/1(in)  "<WiprFront_D_Stat>"
  in/1 -> bus_selector/1

== system test_mdl_NI/CAN_Signal/GWM/SCCM/Steering_Wheel_Data2_FD1_81 ==
  in : Inport
  SelDrvMdeDec_B_RqDrv : Subsystem
  SelDrvMdeInc_B_RqDrv : Subsystem
  SelDrvMdeSwtch_D_Stat4 : Subsystem
  SteEffortInc_B_RqDrv : Subsystem
  SteWhlSwtchBack_B_Stat : Subsystem
  SteWhlSwtchDown_B_Stat : Subsystem
  SteWhlSwtchHome_B_Stat : Subsystem
  SteWhlSwtchHud_B_Stat : Subsystem
  SteWhlSwtchInfo_B_Stat : Subsystem
  SteWhlSwtchIod_B_Stat : Subsystem
  SteWhlSwtchLeft_B_Stat : Subsystem
  SteWhlSwtchMed_B_Stat : Subsystem
  SteWhlSwtchMenu_B_Stat : Subsystem
  SteWhlSwtchNav_B_Stat : Subsystem
  SteWhlSwtchOk_B_Stat : Subsystem
  SteWhlSwtchPhon_B_Stat : Subsystem
  SteWhlSwtchRght_B_Stat : Subsystem
  SteWhlSwtchSet_B_Stat : Subsystem
  SteWhlSwtchUp_B_Stat : Subsystem
  SteWhlSwtchView_B_Stat : Subsystem
  SuspDampInc_B_RqDrv : Subsystem
  bus_creator : BusCreator  Inputs=21
  bus_selector : BusSelector  OutputSignals=SelDrvMdeDec_B_RqDrv,SelDrvMdeInc_B_RqDrv,SelDrvMdeSwtch_D_Stat4,SteEffortInc_B_RqDrv,SteWhlSwtchBack_B_Stat,SteWhlSwtchDown_B_Stat,SteWhlSwtchHome_B_Stat,SteWhlSwtchHud_B_Stat,SteWhlSwtchInfo_B_Stat,SteWhlSwtchIod_B_Stat,SteWhlSwtchLeft_B_Stat,SteWhlSwtchMed_B_Stat,SteWhlSwtchMenu_B_Stat,SteWhlSwtchNav_B_Stat,SteWhlSwtchOk_B_Stat,SteWhlSwtchPhon_B_Stat,SteWhlSwtchRght_B_Stat,SteWhlSwtchSet_B_Stat,SteWhlSwtchUp_B_Stat,SteWhlSwtchView_B_Stat,SuspDampInc_B_RqDrv
  out_port : Outport
  wires:
  bus_creator/1 -> out_port/1  "Steering_Wheel_Data2_FD1_81"
  SelDrvMdeDec_B_RqDrv/1(out) -> bus_creator/1  "SelDrvMdeDec_B_RqDrv"
  SelDrvMdeInc_B_RqDrv/1(out) -> bus_creator/2  "SelDrvMdeInc_B_RqDrv"
  SelDrvMdeSwtch_D_Stat4/1(out) -> bus_creator/3  "SelDrvMdeSwtch_D_Stat4"
  SteEffortInc_B_RqDrv/1(out) -> bus_creator/4  "SteEffortInc_B_RqDrv"
  SteWhlSwtchBack_B_Stat/1(out) -> bus_creator/5  "SteWhlSwtchBack_B_Stat"
  SteWhlSwtchDown_B_Stat/1(out) -> bus_creator/6  "SteWhlSwtchDown_B_Stat"
  SteWhlSwtchHome_B_Stat/1(out) -> bus_creator/7  "SteWhlSwtchHome_B_Stat"
  SteWhlSwtchHud_B_Stat/1(out) -> bus_creator/8  "SteWhlSwtchHud_B_Stat"
  SteWhlSwtchInfo_B_Stat/1(out) -> bus_creator/9  "SteWhlSwtchInfo_B_Stat"
  SteWhlSwtchIod_B_Stat/1(out) -> bus_creator/10  "SteWhlSwtchIod_B_Stat"
  SteWhlSwtchLeft_B_Stat/1(out) -> bus_creator/11  "SteWhlSwtchLeft_B_Stat"
  SteWhlSwtchMed_B_Stat/1(out) -> bus_creator/12  "SteWhlSwtchMed_B_Stat"
  SteWhlSwtchMenu_B_Stat/1(out) -> bus_creator/13  "SteWhlSwtchMenu_B_Stat"
  SteWhlSwtchNav_B_Stat/1(out) -> bus_creator/14  "SteWhlSwtchNav_B_Stat"
  SteWhlSwtchOk_B_Stat/1(out) -> bus_creator/15  "SteWhlSwtchOk_B_Stat"
  SteWhlSwtchPhon_B_Stat/1(out) -> bus_creator/16  "SteWhlSwtchPhon_B_Stat"
  SteWhlSwtchRght_B_Stat/1(out) -> bus_creator/17  "SteWhlSwtchRght_B_Stat"
  SteWhlSwtchSet_B_Stat/1(out) -> bus_creator/18  "SteWhlSwtchSet_B_Stat"
  SteWhlSwtchUp_B_Stat/1(out) -> bus_creator/19  "SteWhlSwtchUp_B_Stat"
  SteWhlSwtchView_B_Stat/1(out) -> bus_creator/20  "SteWhlSwtchView_B_Stat"
  SuspDampInc_B_RqDrv/1(out) -> bus_creator/21  "SuspDampInc_B_RqDrv"
  bus_selector/1 -> SelDrvMdeDec_B_RqDrv/1(in)  "<SelDrvMdeDec_B_RqDrv>"
  bus_selector/2 -> SelDrvMdeInc_B_RqDrv/1(in)  "<SelDrvMdeInc_B_RqDrv>"
  bus_selector/3 -> SelDrvMdeSwtch_D_Stat4/1(in)  "<SelDrvMdeSwtch_D_Stat4>"
  bus_selector/4 -> SteEffortInc_B_RqDrv/1(in)  "<SteEffortInc_B_RqDrv>"
  bus_selector/5 -> SteWhlSwtchBack_B_Stat/1(in)  "<SteWhlSwtchBack_B_Stat>"
  bus_selector/6 -> SteWhlSwtchDown_B_Stat/1(in)  "<SteWhlSwtchDown_B_Stat>"
  bus_selector/7 -> SteWhlSwtchHome_B_Stat/1(in)  "<SteWhlSwtchHome_B_Stat>"
  bus_selector/8 -> SteWhlSwtchHud_B_Stat/1(in)  "<SteWhlSwtchHud_B_Stat>"
  bus_selector/9 -> SteWhlSwtchInfo_B_Stat/1(in)  "<SteWhlSwtchInfo_B_Stat>"
  bus_selector/10 -> SteWhlSwtchIod_B_Stat/1(in)  "<SteWhlSwtchIod_B_Stat>"
  bus_selector/11 -> SteWhlSwtchLeft_B_Stat/1(in)  "<SteWhlSwtchLeft_B_Stat>"
  bus_selector/12 -> SteWhlSwtchMed_B_Stat/1(in)  "<SteWhlSwtchMed_B_Stat>"
  bus_selector/13 -> SteWhlSwtchMenu_B_Stat/1(in)  "<SteWhlSwtchMenu_B_Stat>"
  bus_selector/14 -> SteWhlSwtchNav_B_Stat/1(in)  "<SteWhlSwtchNav_B_Stat>"
  bus_selector/15 -> SteWhlSwtchOk_B_Stat/1(in)  "<SteWhlSwtchOk_B_Stat>"
  bus_selector/16 -> SteWhlSwtchPhon_B_Stat/1(in)  "<SteWhlSwtchPhon_B_Stat>"
  bus_selector/17 -> SteWhlSwtchRght_B_Stat/1(in)  "<SteWhlSwtchRght_B_Stat>"
  bus_selector/18 -> SteWhlSwtchSet_B_Stat/1(in)  "<SteWhlSwtchSet_B_Stat>"
  bus_selector/19 -> SteWhlSwtchUp_B_Stat/1(in)  "<SteWhlSwtchUp_B_Stat>"
  bus_selector/20 -> SteWhlSwtchView_B_Stat/1(in)  "<SteWhlSwtchView_B_Stat>"
  bus_selector/21 -> SuspDampInc_B_RqDrv/1(in)  "<SuspDampInc_B_RqDrv>"
  in/1 -> bus_selector/1

== system test_mdl_NI/CAN_Signal/GWM/Tester_AutoSar/GWM_AutoSar_NetMgmt_FD1 ==
  in : Inport
  GWM_AutoSarNMControl : Subsystem
  GWM_AutoSarNMNodeId : Subsystem
  GWM_AutoSarNMReserved1 : Subsystem
  GWM_AutoSarNMReserved2 : Subsystem
  GWM_AutoSarNMReserved3 : Subsystem
  GWM_AutoSarNMReserved4 : Subsystem
  GWM_GWNMProxy : Subsystem
  GWM_GWOnBoardTester : Subsystem
  bus_creator : BusCreator  Inputs=8
  bus_selector : BusSelector  OutputSignals=GWM_AutoSarNMControl,GWM_AutoSarNMNodeId,GWM_AutoSarNMReserved1,GWM_AutoSarNMReserved2,GWM_AutoSarNMReserved3,GWM_AutoSarNMReserved4,GWM_GWNMProxy,GWM_GWOnBoardTester
  out_port : Outport
  wires:
  bus_creator/1 -> out_port/1  "GWM_AutoSar_NetMgmt_FD1"
  GWM_AutoSarNMControl/1(out) -> bus_creator/1  "GWM_AutoSarNMControl"
  GWM_AutoSarNMNodeId/1(out) -> bus_creator/2  "GWM_AutoSarNMNodeId"
  GWM_AutoSarNMReserved1/1(out) -> bus_creator/3  "GWM_AutoSarNMReserved1"
  GWM_AutoSarNMReserved2/1(out) -> bus_creator/4  "GWM_AutoSarNMReserved2"
  GWM_AutoSarNMReserved3/1(out) -> bus_creator/5  "GWM_AutoSarNMReserved3"
  GWM_AutoSarNMReserved4/1(out) -> bus_creator/6  "GWM_AutoSarNMReserved4"
  GWM_GWNMProxy/1(out) -> bus_creator/7  "GWM_GWNMProxy"
  GWM_GWOnBoardTester/1(out) -> bus_creator/8  "GWM_GWOnBoardTester"
  bus_selector/1 -> GWM_AutoSarNMControl/1(in)  "<GWM_AutoSarNMControl>"
  bus_selector/2 -> GWM_AutoSarNMNodeId/1(in)  "<GWM_AutoSarNMNodeId>"
  bus_selector/3 -> GWM_AutoSarNMReserved1/1(in)  "<GWM_AutoSarNMReserved1>"
  bus_selector/4 -> GWM_AutoSarNMReserved2/1(in)  "<GWM_AutoSarNMReserved2>"
  bus_selector/5 -> GWM_AutoSarNMReserved3/1(in)  "<GWM_AutoSarNMReserved3>"
  bus_selector/6 -> GWM_AutoSarNMReserved4/1(in)  "<GWM_AutoSarNMReserved4>"
  bus_selector/7 -> GWM_GWNMProxy/1(in)  "<GWM_GWNMProxy>"
  bus_selector/8 -> GWM_GWOnBoardTester/1(in)  "<GWM_GWOnBoardTester>"
  in/1 -> bus_selector/1

== system test_mdl_NI/CAN_Signal/GWM/Tester_AutoSar/TesterPhysicalResGWM_FD1 ==
  in : Inport
  TesterPhysicalResGWM_F1 : Subsystem
  bus_creator : BusCreator  Inputs=1
  bus_selector : BusSelector  OutputSignals=TesterPhysicalResGWM_F1
  out_port : Outport
  wires:
  bus_creator/1 -> out_port/1  "TesterPhysicalResGWM_FD1"
  TesterPhysicalResGWM_F1/1(out) -> bus_creator/1  "TesterPhysicalResGWM_F1"
  bus_selector/1 -> TesterPhysicalResGWM_F1/1(in)  "<TesterPhysicalResGWM_F1>"
  in/1 -> bus_selector/1

== system test_mdl_NI/CAN_Signal/PSCM/EPAS_INFO_0x82/DrvSteActv_B_Stat ==
  in : Inport
  out : Outport
  wires:
  in/1 -> out/1

== system test_mdl_NI/CAN_Signal/PSCM/EPAS_INFO_0x82/DrvSte_Tq_Actl ==
  in : Inport
  out : Outport
  wires:
  in/1 -> out/1

== system test_mdl_NI/CAN_Signal/PSCM/EPAS_INFO_0x82/EPAS_Failure ==
  in : Inport
  out : Outport
  wires:
  in/1 -> out/1

== system test_mdl_NI/CAN_Signal/PSCM/EPAS_INFO_0x82/SAPPAngleControlStat1 ==
  in : Inport
  out : Outport
  wires:
  in/1 -> out/1

== system test_mdl_NI/CAN_Signal/PSCM/EPAS_INFO_0x82/SAPPAngleControlStat2 ==
  in : Inport
  out : Outport
  wires:
  in/1 -> out/1

== system test_mdl_NI/CAN_Signal/PSCM/EPAS_INFO_0x82/SAPPAngleControlStat3 ==
  in : Inport
  out : Outport
  wires:
  in/1 -> out/1

== system test_mdl_NI/CAN_Signal/PSCM/EPAS_INFO_0x82/SAPPAngleControlStat4 ==
  in : Inport
  out : Outport
  wires:
  in/1 -> out/1

== system test_mdl_NI/CAN_Signal/PSCM/EPAS_INFO_0x82/SAPPAngleControlStat5 ==
  in : Inport
  out : Outport
  wires:
  in/1 -> out/1

== system test_mdl_NI/CAN_Signal/PSCM/EPAS_INFO_0x82/SAPPAngleControlStat6 ==
  in : Inport
  out : Outport
  wires:
  in/1 -> out/1

== system test_mdl_NI/CAN_Signal/PSCM/EPAS_INFO_0x82/SteMdule_D_Stat ==
  in : Inport
  out : Outport
  wires:
  in/1 -> out/1

== system test_mdl_NI/CAN_Signal/PSCM/EPAS_INFO_0x82/SteMdule_I_Est ==
  in : Inport
  out : Outport
  wires:
  in/1 -> out/1

== system test_mdl_NI/CAN_Signal/PSCM/EPAS_INFO_0x82/SteMdule_U_Meas ==
  in : Inport
  out : Outport
  wires:
  in/1 -> out/1

== system test_mdl_NI/CAN_Signal/PSCM/EPAS_INFO_0x82/SteeringColumnTorque ==
  in : Inport
  out : Outport
  wires:
  in/1 -> out/1

== system test_mdl_NI/CAN_Signal/PSCM/EPAS_INFO_0x82/TrlrHitchLamp_D_Rqst ==
  in : Inport
  out : Outport
  wires:
  in/1 -> out/1

== system test_mdl_NI/CAN_Signal/PSCM/EPAS_INFO_0x82/VehVTrlrAid_B_Rq ==
  in : Inport
  out : Outport
  wires:
  in/1 -> out/1

== system test_mdl_NI/CAN_Signal/PSCM/EPAS_INFO_0x82/Veh_V_RqMxTrlrAid ==
  in : Inport
  out : Outport
  wires:
  in/1 -> out/1

== system test_mdl_NI/CAN_Signal/PSCM/Lane_Assist_Data3_FD1_0x3CC/LaActAvail_D_Actl ==
  in : Inport
  out : Outport
  wires:
  in/1 -> out/1

== system test_mdl_NI/CAN_Signal/PSCM/Lane_Assist_Data3_FD1_0x3CC/LaActDeny_B_Actl ==
  in : Inport
  out : Outport
  wires:
  in/1 -> out/1

== system test_mdl_NI/CAN_Signal/PSCM/Lane_Assist_Data3_FD1_0x3CC/LaHandsOff_B_Actl ==
  in : Inport
  out : Outport
  wires:
  in/1 -> out/1

== system test_mdl_NI/CAN_Signal/PSCM/Lane_Assist_Data3_FD1_0x3CC/LsmcBrkDecelEnbl_D_Rq ==
  in : Inport
  out : Outport
  wires:
  in/1 -> out/1

== system test_mdl_NI/CAN_Signal/PSCM/Lane_Assist_Data3_FD1_0x3CC/LsmcBrk_Tq_Rq ==
  in : Inport
  out : Outport
  wires:
  in/1 -> out/1

== system test_mdl_NI/CAN_Signal/PSCM/Lane_Assist_Data3_FD1_0x3CC/TjaHandsOnCnfdnc_B_Est ==
  in : Inport
  out : Outport
  wires:
  in/1 -> out/1

== system test_mdl_NI/CAN_Signal/PSCM/Lane_Assist_Data3_FD1_0x3CC/TrlrAn_An_TrgtCalc ==
  in : Inport
  out : Outport
  wires:
  in/1 -> out/1

== system test_mdl_NI/CAN_Signal/PSCM/PSCM_AutoSar_NetwrkMgmt_0x5B5/PSCM_AutoSarNMControl ==
  in : Inport
  out : Outport
  wires:
  in/1 -> out/1

== system test_mdl_NI/CAN_Signal/PSCM/PSCM_AutoSar_NetwrkMgmt_0x5B5/PSCM_AutoSarNMNodeId ==
  in : Inport
  out : Outport
  wires:
  in/1 -> out/1

== system test_mdl_NI/CAN_Signal/PSCM/PSCM_AutoSar_NetwrkMgmt_0x5B5/PSCM_AutoSarNMReserved1 ==
  in : Inport
  out : Outport
  wires:
  in/1 -> out/1

== system test_mdl_NI/CAN_Signal/PSCM/PSCM_AutoSar_NetwrkMgmt_0x5B5/PSCM_AutoSarNMReserved2 ==
  in : Inport
  out : Outport
  wires:
  in/1 -> out/1

== system test_mdl_NI/CAN_Signal/PSCM/PSCM_AutoSar_NetwrkMgmt_0x5B5/PSCM_AutoSarNMReserved3 ==
  in : Inport
  out : Outport
  wires:
  in/1 -> out/1

== system test_mdl_NI/CAN_Signal/PSCM/PSCM_AutoSar_NetwrkMgmt_0x5B5/PSCM_AutoSarNMReserved4 ==
  in : Inport
  out : Outport
  wires:
  in/1 -> out/1

== system test_mdl_NI/CAN_Signal/PSCM/PSCM_AutoSar_NetwrkMgmt_0x5B5/PSCM_GWNMProxy ==
  in : Inport
  out : Outport
  wires:
  in/1 -> out/1

== system test_mdl_NI/CAN_Signal/PSCM/PSCM_AutoSar_NetwrkMgmt_0x5B5/PSCM_GWOnBoardTester ==
  in : Inport
  out : Outport
  wires:
  in/1 -> out/1

== system test_mdl_NI/CAN_Signal/PSCM/SteeringPinion_Data_0x7E/StePinAn_No_Cnt ==
  in : Inport
  out : Outport
  wires:
  in/1 -> out/1

== system test_mdl_NI/CAN_Signal/PSCM/SteeringPinion_Data_0x7E/StePinAn_No_Cs ==
  in : Inport
  out : Outport
  wires:
  in/1 -> out/1

== system test_mdl_NI/CAN_Signal/PSCM/SteeringPinion_Data_0x7E/StePinCompAnEst_D_Qf ==
  in : Inport
  out : Outport
  wires:
  in/1 -> out/1

== system test_mdl_NI/CAN_Signal/PSCM/SteeringPinion_Data_0x7E/StePinComp_An_Est ==
  in : Inport
  out : Outport
  wires:
  in/1 -> out/1

== system test_mdl_NI/CAN_Signal/PSCM/SteeringPinion_Data_0x7E/StePinRelInit_An_Sns ==
  in : Inport
  out : Outport
  wires:
  in/1 -> out/1

== system test_mdl_NI/CAN_Signal/PSCM/SteeringPinion_Data_0x7E/StePw_B_Rq ==
  in : Inport
  out : Outport
  wires:
  in/1 -> out/1

== system test_mdl_NI/CAN_Signal/PSCM/TesterPhysicalResPSCM_0x738/TesterPhysicalResPSCM ==
  in : Inport
  out : Outport
  wires:
  in/1 -> out/1

== system test_mdl_NI/CAN_Signal/PSCM/TrailerAid_Data2_0x417/EsaOn_B_Stat ==
  in : Inport
  out : Outport
  wires:
  in/1 -> out/1

== system test_mdl_NI/CAN_Signal/PSCM/TrailerAid_Data2_0x417/HitchToTrlrAxle_L_Calc ==
  in : Inport
  out : Outport
  wires:
  in/1 -> out/1

== system test_mdl_NI/CAN_Signal/PSCM/TrailerAid_Data2_0x417/LatCtlLim_D_Stat ==
  in : Inport
  out : Outport
  wires:
  in/1 -> out/1

== system test_mdl_NI/CAN_Signal/PSCM/TrailerAid_Data2_0x417/LatCtlSte_D_Stat ==
  in : Inport
  out : Outport
  wires:
  in/1 -> out/1

== system test_mdl_NI/CAN_Signal/PSCM/TrailerAid_Data2_0x417/SelDrvMdeSte_D_Stat ==
  in : Inport
  out : Outport
  wires:
  in/1 -> out/1

== system test_mdl_NI/CAN_Signal/PSCM/TrailerAid_Data2_0x417/TrlrAidEnbl_D2_Stat ==
  in : Inport
  out : Outport
  wires:
  in/1 -> out/1

== system test_mdl_NI/CAN_Signal/PSCM/TrailerAid_Data2_0x417/TrlrAidMsgTxt_D2_Rq ==
  in : Inport
  out : Outport
  wires:
  in/1 -> out/1

== system test_mdl_NI/CAN_Signal/PSCM/TrailerAid_Data2_0x417/TrlrAidSetup_D2_Stat ==
  in : Inport
  out : Outport
  wires:
  in/1 -> out/1

== system test_mdl_NI/CAN_Signal/PSCM/TrailerAid_Data2_0x417/TrlrAidTrgtId_No_Rq ==
  in : Inport
  out : Outport
  wires:
  in/1 -> out/1

== system test_mdl_NI/CAN_Signal/PSCM/TrailerAid_Data2_0x417/TrlrAidTrlrId_No_Rq ==
  in : Inport
  out : Outport
  wires:
  in/1 -> out/1

== system test_mdl_NI/CAN_Signal/PSCM/TrailerAid_Data2_0x417/TrlrAnOffst_An2_Calc ==
  in : Inport
  out : Outport
  wires:
  in/1 -> out/1

== system test_mdl_NI/CAN_Signal/PSCM/TrailerAid_Data2_0x417/TrlrAn_An_MxCalc ==
  in : Inport
  out : Outport
  wires:
  in/1 -> out/1

== system test_mdl_NI/CAN_Signal/PSCM/TrailerAid_Data2_0x417/TrlrAn_An_WarnCalc ==
  in : Inport
  out : Outport
  wires:
  in/1 -> out/1

== system test_mdl_NI/CAN_Signal/RealPCM/EngBrakeData/CcStat_D_Actl ==
  in : Inport
  out : Outport
  wires:
  in/1 -> out/1

== system test_mdl_NI/CAN_Signal/RealPCM/EngVehicleSpThrottle2/Veh_V_ActlEng ==
  in : Inport
  out : Outport
  wires:
  in/1 -> out/1

== system test_mdl_NI/CAN_Signal/RealPCM/user_channel/Desired_Speed ==
  in : Inport
  out : Outport
  wires:
  in/1 -> out/1

== system test_mdl_NI/CAN_Signal/RealPCM/user_channel/PCM_status_user_input ==
  in : Inport
  out : Outport
  wires:
  in/1 -> out/1

== system test_mdl_NI/To_NI_HIL/DSMC/DrvStatMonData/DrvEngLvlConfid_D_Stat ==
  in : Inport
  out : Outport
  wires:
  in/1 -> out/1

== system test_mdl_NI/To_NI_HIL/DSMC/DrvStatMonData/DrvEngageLevel_No_Cnt ==
  in : Inport
  out : Outport
  wires:
  in/1 -> out/1

== system test_mdl_NI/To_NI_HIL/DSMC/DrvStatMonData/DrvEngageLevel_No_Cs ==
  in : Inport
  out : Outport
  wires:
  in/1 -> out/1

== system test_mdl_NI/To_NI_HIL/SRR_L/FL_SOD/SRR_FL_001 ==
  in : Inport
  SRR_FL_CAN_DET_AMPLITUDE_01 : Subsystem
  SRR_FL_CAN_DET_AZIMUTH_01 : Subsystem
  SRR_FL_CAN_DET_ELEVATION_01 : Subsystem
  SRR_FL_CAN_DET_RANGE_01 : Subsystem
  SRR_FL_CAN_DET_RANGE_RATE_01 : Subsystem
  SRR_FL_CAN_DET_SUPER_RES_TARGET_01 : Subsystem
  SRR_FL_CAN_DET_VALID_LEVEL_01 : Subsystem
  bus_creator : BusCreator  Inputs=7
  bus_selector : BusSelector  OutputSignals=SRR_FL_CAN_DET_RANGE_01,SRR_FL_CAN_DET_RANGE_RATE_01,SRR_FL_CAN_DET_AZIMUTH_01,SRR_FL_CAN_DET_ELEVATION_01,SRR_FL_CAN_DET_SUPER_RES_TARGET_01,SRR_FL_CAN_DET_AMPLITUDE_01,SRR_FL_CAN_DET_VALID_LEVEL_01
  out_port : Outport
  wires:
  bus_creator/1 -> out_port/1  "SRR_FL_001"
  SRR_FL_CAN_DET_RANGE_01/1(out) -> bus_creator/1  "SRR_FL_CAN_DET_RANGE_01"
  SRR_FL_CAN_DET_RANGE_RATE_01/1(out) -> bus_creator/2  "SRR_FL_CAN_DET_RANGE_RATE_01"
  SRR_FL_CAN_DET_AZIMUTH_01/1(out) -> bus_creator/3  "SRR_FL_CAN_DET_AZIMUTH_01"
  SRR_FL_CAN_DET_ELEVATION_01/1(out) -> bus_creator/4  "SRR_FL_CAN_DET_ELEVATION_01"
  SRR_FL_CAN_DET_SUPER_RES_TARGET_01/1(out) -> bus_creator/5  "SRR_FL_CAN_DET_SUPER_RES_TARGET_01"
  SRR_FL_CAN_DET_AMPLITUDE_01/1(out) -> bus_creator/6  "SRR_FL_CAN_DET_AMPLITUDE_01"
  SRR_FL_CAN_DET_VALID_LEVEL_01/1(out) -> bus_creator/7  "SRR_FL_CAN_DET_VALID_LEVEL_01"
  bus_selector/1 -> SRR_FL_CAN_DET_RANGE_01/1(in)  "<SRR_FL_CAN_DET_RANGE_01>"
  bus_selector/2 -> SRR_FL_CAN_DET_RANGE_RATE_01/1(in)  "<SRR_FL_CAN_DET_RANGE_RATE_01>"
  bus_selector/3 -> SRR_FL_CAN_DET_AZIMUTH_01/1(in)  "<SRR_FL_CAN_DET_AZIMUTH_01>"
  bus_selector/4 -> SRR_FL_CAN_DET_ELEVATION_01/1(in)  "<SRR_FL_CAN_DET_ELEVATION_01>"
  bus_selector/5 -> SRR_FL_CAN_DET_SUPER_RES_TARGET_01/1(in)  "<SRR_FL_CAN_DET_SUPER_RES_TARGET_01>"
  bus_selector/6 -> SRR_FL_CAN_DET_AMPLITUDE_01/1(in)  "<SRR_FL_CAN_DET_AMPLITUDE_01>"
  bus_selector/7 -> SRR_FL_CAN_DET_VALID_LEVEL_01/1(in)  "<SRR_FL_CAN_DET_VALID_LEVEL_01>"
  in/1 -> bus_selector/1

== system test_mdl_NI/To_NI_HIL/SRR_L/FL_SOD/SRR_FL_002 ==
  in : Inport
  SRR_FL_CAN_DET_AMPLITUDE_02 : Subsystem
  SRR_FL_CAN_DET_AZIMUTH_02 : Subsystem
  SRR_FL_CAN_DET_ELEVATION_02 : Subsystem
  SRR_FL_CAN_DET_RANGE_02 : Subsystem
  SRR_FL_CAN_DET_RANGE_RATE_02 : Subsystem
  SRR_FL_CAN_DET_SUPER_RES_TARGET_02 : Subsystem
  SRR_FL_CAN_DET_VALID_LEVEL_02 : Subsystem
  bus_creator : BusCreator  Inputs=7
  bus_selector : BusSelector  OutputSignals=SRR_FL_CAN_DET_RANGE_02,SRR_FL_CAN_DET_RANGE_RATE_02,SRR_FL_CAN_DET_AZIMUTH_02,SRR_FL_CAN_DET_ELEVATION_02,SRR_FL_CAN_DET_SUPER_RES_TARGET_02,SRR_FL_CAN_DET_AMPLITUDE_02,SRR_FL_CAN_DET_VALID_LEVEL_02
  out_port : Outport
  wires:
  bus_creator/1 -> out_port/1  "SRR_FL_002"
  SRR_FL_CAN_DET_RANGE_02/1(out) -> bus_creator/1  "SRR_FL_CAN_DET_RANGE_02"
  SRR_FL_CAN_DET_RANGE_RATE_02/1(out) -> bus_creator/2  "SRR_FL_CAN_DET_RANGE_RATE_02"
  SRR_FL_CAN_DET_AZIMUTH_02/1(out) -> bus_creator/3  "SRR_FL_CAN_DET_AZIMUTH_02"
  SRR_FL_CAN_DET_ELEVATION_02/1(out) -> bus_creator/4  "SRR_FL_CAN_DET_ELEVATION_02"
  SRR_FL_CAN_DET_SUPER_RES_TARGET_02/1(out) -> bus_creator/5  "SRR_FL_CAN_DET_SUPER_RES_TARGET_02"
  SRR_FL_CAN_DET_AMPLITUDE_02/1(out) -> bus_creator/6  "SRR_FL_CAN_DET_AMPLITUDE_02"
  SRR_FL_CAN_DET_VALID_LEVEL_02/1(out) -> bus_creator/7  "SRR_FL_CAN_DET_VALID_LEVEL_02"
  bus_selector/1 -> SRR_FL_CAN_DET_RANGE_02/1(in)  "<SRR_FL_CAN_DET_RANGE_02>"
  bus_selector/2 -> SRR_FL_CAN_DET_RANGE_RATE_02/1(in)  "<SRR_FL_CAN_DET_RANGE_RATE_02>"
  bus_selector/3 -> SRR_FL_CAN_DET_AZIMUTH_02/1(in)  "<SRR_FL_CAN_DET_AZIMUTH_02>"
  bus_selector/4 -> SRR_FL_CAN_DET_ELEVATION_02/1(in)  "<SRR_FL_CAN_DET_ELEVATION_02>"
  bus_selector/5 -> SRR_FL_CAN_DET_SUPER_RES_TARGET_02/1(in)  "<SRR_FL_CAN_DET_SUPER_RES_TARGET_02>"
  bus_selector/6 -> SRR_FL_CAN_DET_AMPLITUDE_02/1(in)  "<SRR_FL_CAN_DET_AMPLITUDE_02>"
  bus_selector/7 -> SRR_FL_CAN_DET_VALID_LEVEL_02/1(in)  "<SRR_FL_CAN_DET_VALID_LEVEL_02>"
  in/1 -> bus_selector/1

== system test_mdl_NI/To_NI_HIL/SRR_L/FL_SOD/SRR_FL_003 ==
  in : Inport
  SRR_FL_CAN_DET_AMPLITUDE_03 : Subsystem
  SRR_FL_CAN_DET_AZIMUTH_03 : Subsystem
  SRR_FL_CAN_DET_ELEVATION_03 : Subsystem
  SRR_FL_CAN_DET_RANGE_03 : Subsystem
  SRR_FL_CAN_DET_RANGE_RATE_03 : Subsystem
  SRR_FL_CAN_DET_SUPER_RES_TARGET_03 : Subsystem
  SRR_FL_CAN_DET_VALID_LEVEL_03 : Subsystem
  bus_creator : BusCreator  Inputs=7
  bus_selector : BusSelector  OutputSignals=SRR_FL_CAN_DET_RANGE_03,SRR_FL_CAN_DET_RANGE_RATE_03,SRR_FL_CAN_DET_AZIMUTH_03,SRR_FL_CAN_DET_ELEVATION_03,SRR_FL_CAN_DET_SUPER_RES_TARGET_03,SRR_FL_CAN_DET_AMPLITUDE_03,SRR_FL_CAN_DET_VALID_LEVEL_03
  out_port : Outport
  wires:
  bus_creator/1 -> out_port/1  "SRR_FL_003"
  SRR_FL_CAN_DET_RANGE_03/1(out) -> bus_creator/1  "SRR_FL_CAN_DET_RANGE_03"
  SRR_FL_CAN_DET_RANGE_RATE_03/1(out) -> bus_creator/2  "SRR_FL_CAN_DET_RANGE_RATE_03"
  SRR_FL_CAN_DET_AZIMUTH_03/1(out) -> bus_creator/3  "SRR_FL_CAN_DET_AZIMUTH_03"
  SRR_FL_CAN_DET_ELEVATION_03/1(out) -> bus_creator/4  "SRR_FL_CAN_DET_ELEVATION_03"
  SRR_FL_CAN_DET_SUPER_RES_TARGET_03/1(out) -> bus_creator/5  "SRR_FL_CAN_DET_SUPER_RES_TARGET_03"
  SRR_FL_CAN_DET_AMPLITUDE_03/1(out) -> bus_creator/6  "SRR_FL_CAN_DET_AMPLITUDE_03"
  SRR_FL_CAN_DET_VALID_LEVEL_03/1(out) -> bus_creator/7  "SRR_FL_CAN_DET_VALID_LEVEL_03"
  bus_selector/1 -> SRR_FL_CAN_DET_RANGE_03/1(in)  "<SRR_FL_CAN_DET_RANGE_03>"
  bus_selector/2 -> SRR_FL_CAN_DET_RANGE_RATE_03/1(in)  "<SRR_FL_CAN_DET_RANGE_RATE_03>"
  bus_selector/3 -> SRR_FL_CAN_DET_AZIMUTH_03/1(in)  "<SRR_FL_CAN_DET_AZIMUTH_03>"
  bus_selector/4 -> SRR_FL_CAN_DET_ELEVATION_03/1(in)  "<SRR_FL_CAN_DET_ELEVATION_03>"
  bus_selector/5 -> SRR_FL_CAN_DET_SUPER_RES_TARGET_03/1(in)  "<SRR_FL_CAN_DET_SUPER_RES_TARGET_03>"
  bus_selector/6 -> SRR_FL_CAN_DET_AMPLITUDE_03/1(in)  "<SRR_FL_CAN_DET_AMPLITUDE_03>"
  bus_selector/7 -> SRR_FL_CAN_DET_VALID_LEVEL_03/1(in)  "<SRR_FL_CAN_DET_VALID_LEVEL_03>"
  in/1 -> bus_selector/1
